simulink model "hisf_0002_User_specified_state_transition_execution_order"  (R2018b)
settings: Solver=VariableStepAuto  StartTime=0.0  StopTime=10.0  RelTol=1e-3
model workspace (MAT data in the model file):
  Iei = 0.0219914882836
  converter_data = [0  137.465208994  2.232; 0.1  137.065019157  2.075; 0.2  135.864449646  1.975; 0.3  135.664354728  1.846; 0.4  137.565256453  1.72; 0.5  140.366585312  1.564; 0.6  145.268910814  1.409; 0.7  152.872517717  1.254; 0.8  162.9773111  1.096; 0.81  164.27792807  1.08; 0.82  166.178829795  1.061; 0.83  167.979684062  1.043; 0.84  170.080680706  1.028; 0.85  172.781962105  1.012; 0.86  175.383196045  1.002; 0.87  179.585189333  1.002; 0.88  183.587087703  1.001; 0.89  189.890077635  0.998; 0.9  197.693779455  0.999; 0.92  215.902417037  1.001; 0.94  244.515990379  1.002]
  downtab = [0  5  20  35; 0  5  20  35; 0  5  25  40; 0  5  30  50; 0  30  50  80; 0  30  50  80]
  downth = [0; 5; 40; 50; 90; 100]
  emap = [-40  -44  -49  -53  -57  -61  -65  -70  -74  -78  -82; 215  117  85  66  44  29  10  -2  -13  -22  -32; 245  208  178  148  122  104  85  66  48  33  18; 264  260  241  219  193  167  152  133  119  96  85; 264  279  282  275  260  238  223  208  189  171  152; 267  290  293  297  290  275  260  256  234  212  193; 267  297  305  305  305  301  293  282  267  249  226; 267  301  308  312  319  323  319  316  297  279  253; 267  301  312  319  327  327  327  327  312  293  267; 267  301  312  319  327  334  334  334  319  305  275]
  nevec = [800 1200 1600 2000 2400 2800 3200 3600 4000 4400 4800]
  p0 = 0.07934
  p1 = 0.07934
  thvec = [0; 20; 30; 40; 50; 60; 70; 80; 90; 100]
  uptab = [10  30  50  1000000; 10  30  50  1000000; 15  30  50  1000000; 23  41  60  1000000; 40  70  100  1000000; 40  70  100  1000000]
  upth = [0; 25; 35; 50; 90; 100]
  vehicledata = [3.23; 40; 0.3; 1; 50; 0]
settings Model: Creator=amyyang  LastModifiedBy=amyyang

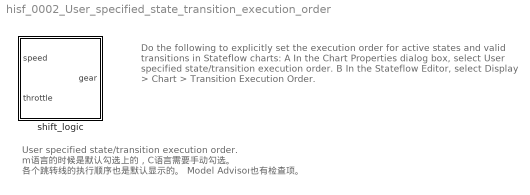
== system hisf_0002_User_specified_state_transition_execution_order ==
  note: User specified state/transition execution order. m语言的时候是默认勾选上的，C语言需要手动勾选。
      | 各个跳转线的执行顺序也是默认显示的。
      |
      | Model Advisor也有检查项。
  note: Do the following to explicitly set the execution order for active states and valid
      | transitions in Stateflow charts:
      | A In the Chart Properties dialog box, select User specified state/transition
      | execution order.
      | B In the Stateflow Editor, select Display > Chart > Transition Execution
      | Order.
  shift_logic : Stateflow chart  TreatAsAtomicUnit=on  mask{TWAIT=2}
      mask prompts: TWAIT "Delay before gear change (tick)"

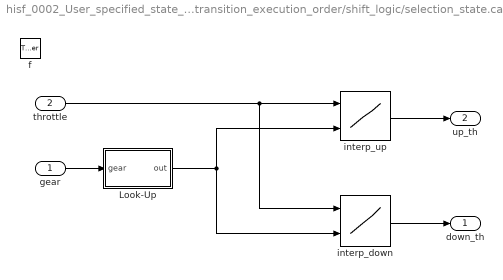
== system hisf_0002_User_specified_state_transition_execution_order/shift_logic/selection_state.calc_th ==
  gear : Inport  OutDataTypeStr=Enum: gearType  PortDimensions=1
  throttle : Inport  Port=2  OutDataTypeStr=double  PortDimensions=1
  f : TriggerPort  TriggerType=function-call  VariantControl=Variant
      settings: CopyFcn=Stateflow.SLINSF.SimulinkMan.removeBlockPreDeleteFcn  PreDeleteFcn=Stateflow.SLINSF.SimulinkMan.unsafePredeleteFcn
  Look-Up : MATLAB Function  TreatAsAtomicUnit=on
  interp_down : Lookup_n-D  BreakpointsForDimension1=downth  BreakpointsForDimension2=[1:4]  Table=downtab  InputSameDT=on
  interp_up : Lookup_n-D  BreakpointsForDimension1=upth  BreakpointsForDimension2=[1:4]  Table=uptab  InputSameDT=on
  down_th : Outport
  up_th : Outport  Port=2
  wires:
  Look-Up/1(out) -> interp_up/2, interp_down/2
  gear/1 -> Look-Up/1(gear)
  throttle/1 -> interp_up/1, interp_down/1
  interp_down/1 -> down_th/1
  interp_up/1 -> up_th/1

== stateflow chart hisf_0002_User_specified_state_transition_execution_order/shift_logic ==
  settings: updateMethod=DISCRETE  sampleTime=0.04
  state gear_state [parallel]
    settings: executionOrder=1
    state fourth
    state third
    state second
    state first
    (default) -> first
    second -> third [order 1] : UP
    third -> fourth [order 1] : UP
    first -> second : UP
    fourth -> third : DOWN
    third -> second [order 2] : DOWN
    second -> first [order 2] : DOWN
  state selection_state [parallel]
    during: [down_th,up_th] = calc_th(gear,throttle);
    settings: executionOrder=2
    state steady_state
    state upshifting
    state downshifting
    state [down_th,up_th] = calc_th(gear,throttle) [function]
    (default) -> steady_state
    steady_state -> upshifting [order 1] : [speed > up_th]
    steady_state -> downshifting [order 2] : [speed < down_th]
    downshifting -> steady_state [order 1] : after(TWAIT,tick)
        | [speed <= down_th]
        | {send(gear_state.DOWN)}
    downshifting -> steady_state [order 2] : [speed > down_th]
    upshifting -> steady_state [order 1] : after(TWAIT,tick)
        | [speed >= up_th]
        | {send(gear_state.UP)}
    upshifting -> steady_state [order 2] : [speed < up_th]
  data: gear function_input Enum: gearType size=1; throttle function_input double size=1; down_th function_output; up_th function_output; speed input double; TWAIT parameter uint8; up_th local double; down_th local double; throttle input; gear output Enum: gearType
  events: DOWN local EITHER_EDGE_EVENT; UP local EITHER_EDGE_EVENT

== matlab function hisf_0002_User_specified_state_transition_execution_order/shift_logic/selection_state.calc_th/Look-Up ==
  data: gear input; out output
function out = fcn(gear)
    %#codegen
    table = [1 2 3 4];
    switch(gear)
        case gearType.fourth;
            out=table(4);        
        case gearType.third;
            out=table(3);
        case gearType.second;
            out=table(2);            
        otherwise; % gearType.first
            out=table(1);
    end
    
end
